simulink model "pt8612pll_2"  (Simulink 5.0)
settings: Solver=ode45  StartTime=0.0  StopTime=100  RelTol=1e-8  AbsTol=1e-11
values from neighbouring files (symbols this model uses):
  C = 680e-9    (= 6.8e-07)    [PT8612PLLinit.m]    (also in PT8612PLLinit_2.m; PT8612PLLinit_3.m; PT8612PLLinit_4.m; colorimetry_rom.m = [[CrCgCb(1) 0 0];[0 CrCgCb(2) 0];[0 0 CrCgCb(3)]])
  fvcxo = 148.5e6/1.001    (= 148351648.352)    [PT8612PLLinit.m]    (also in PT8612PLLinit_2.m; PT8612PLLinit_3.m; PT8612PLLinit_4.m)
  Gi = 1/32    (= 0.03125)    [PT8612PLLinit.m]    (also in PT8612PLLinit_2.m = 0.05)
  Gp = 1/4    (= 0.25)    [PT8612PLLinit.m]    (also in PT8612PLLinit_2.m = 0.025; PT8612PLLinit_4.m = 256)
  Kvcxo = 90e-6    (= 9e-05)    [PT8612PLLinit.m]    (also in PT8612PLLinit_2.m; PT8612PLLinit_3.m; PT8612PLLinit_4.m)
  Nbit = 12    [PT8612PLLinit_2.m]    (also in PT8612PLLinit_3.m)
  R = 100e3    (= 100000)    [PT8612PLLinit.m]    (also in PT8612PLLinit_2.m = 220000; PT8612PLLinit_3.m = 82000; PT8612PLLinit_4.m = 200000; combi_signal.m = [R;ones(red_heigth,spl)])
  Tds = 8/fvcxo    (= 5.39259259259e-08)    [PT8612PLLinit_2.m]    (also in PT8612PLLinit_3.m; PT8612PLLinit_4.m)
  Vcc = 3.3    [PT8612PLLinit_2.m]    (also in PT8612PLLinit_3.m; PT8612PLLinit_4.m)
libraries: simulink x2
settings Model: LastModifiedBy=thh

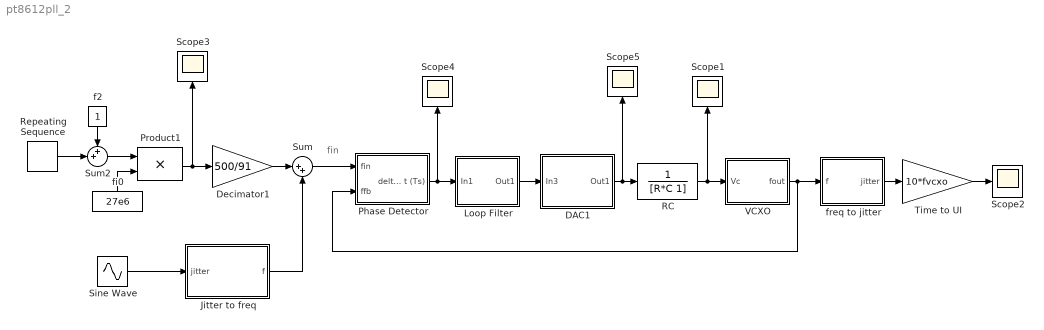
== system pt8612pll_2 ==
  note: fin
  DAC1 : Subsystem
  Decimator1 : Gain  Gain=500/91  SaturateOnIntegerOverflow=on
  Jitter to freq : Subsystem
  Loop Filter : Subsystem
  Phase Detector : Subsystem
  Product1 : Product  SaturateOnIntegerOverflow=on
  RC : TransferFcn  Denominator=[R*C 1]
  Repeating Sequence : simulink/Sources/Repeating Sequence  rep_seq_t=[0 1 1 1000]  rep_seq_y=[1 1 0 0]*1e-9
  Scope{1..5} (5 alike) : Scope
      Scope1 settings: Orientation=up  TimeRange=10  YMin=-0.35  YMax=0.2
      Scope2 settings: TimeRange=10  YMin=1.48  YMax=1.56  SaveName=ScopeData3
      Scope3 settings: Orientation=up  YMin=5.55112e-017  YMax=1.9  SaveName=ScopeData4
      Scope4 settings: Orientation=up  TimeRange=10  YMin=-0.5  YMax=0.5
      Scope5 settings: Orientation=up  TimeRange=10  YMin=-0.35  YMax=0.2  SaveName=ScopeData5
  Sine Wave : Sin  Amplitude=1e-9  Frequency=100  SampleTime=0
  Sum : Sum  Inputs=|++  SaturateOnIntegerOverflow=on
  Sum2 : Sum  Inputs=++|  SaturateOnIntegerOverflow=on
  Time to UI : Gain  Gain=10*fvcxo  SaturateOnIntegerOverflow=on
  VCXO : Subsystem
  f2 : Constant  Orientation=down
  fi0 : Constant  Orientation=up  Value=27e6
  freq to jitter : Subsystem
  wires:
  Phase Detector/1(delta t (Ts)) -> Loop Filter/1(In1), Scope4/1
  VCXO/1(fout) -> freq to jitter/1(f), Phase Detector/2(ffb)
  Product1/1 -> Scope3/1, Decimator1/1
  f2/1 -> Sum2/1
  Sum2/1 -> Product1/1
  Repeating Sequence/1 -> Sum2/2
  Loop Filter/1(Out1) -> DAC1/1(In3)
  freq to jitter/1(jitter) -> Time to UI/1
  fi0/1 -> Product1/2
  Time to UI/1 -> Scope2/1
  Sum/1 -> Phase Detector/1(fin)
  Decimator1/1 -> Sum/1
  Jitter to freq/1(f) -> Sum/2
  Sine Wave/1 -> Jitter to freq/1(jitter)
  DAC1/1(Out1) -> RC/1, Scope5/1
  RC/1 -> VCXO/1(Vc), Scope1/1

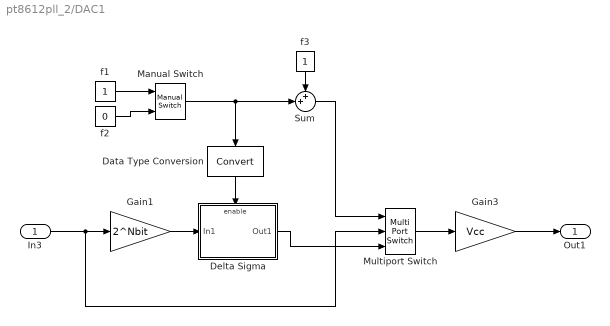
== system pt8612pll_2/DAC1 ==
  In3 : Inport
  Data Type Conversion : DataTypeConversion  Orientation=down  DataType=boolean  SaturateOnIntegerOverflow=on
  Delta Sigma : Subsystem
  Gain1 : Gain  Gain=2^Nbit  SaturateOnIntegerOverflow=on
  Gain3 : Gain  Gain=Vcc  SaturateOnIntegerOverflow=on
  Manual Switch : simulink/Signal Routing/Manual Switch  sw=0  action=0
  Multiport Switch : MultiPortSwitch  Inputs=2  SaturateOnIntegerOverflow=on
  Sum : Sum  Inputs=++|  SaturateOnIntegerOverflow=on
  f1 : Constant
  f2 : Constant  Value=0
  f3 : Constant  Orientation=down
  Out1 : Outport
  wires:
  Delta Sigma/1(Out1) -> Multiport Switch/3
  f3/1 -> Sum/1
  Sum/1 -> Multiport Switch/1
  Gain3/1 -> Out1/1
  Gain1/1 -> Delta Sigma/1(In1)
  Multiport Switch/1 -> Gain3/1
  f2/1 -> Manual Switch/2
  f1/1 -> Manual Switch/1
  Manual Switch/1 -> Sum/2, Data Type Conversion/1
  In3/1 -> Multiport Switch/2, Gain1/1
  Data Type Conversion/1 -> Delta Sigma/Enable

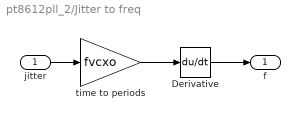
== system pt8612pll_2/Jitter to freq ==
  jitter : Inport
  Derivative : Derivative
  time to periods : Gain  Gain=fvcxo  SaturateOnIntegerOverflow=on
  f : Outport
  wires:
  time to periods/1 -> Derivative/1
  jitter/1 -> time to periods/1
  Derivative/1 -> f/1

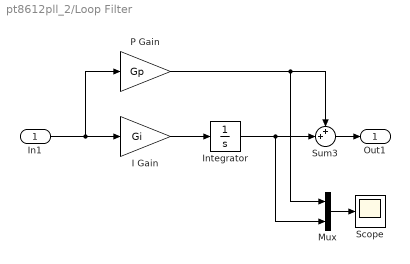
== system pt8612pll_2/Loop Filter ==
  In1 : Inport
  I Gain : Gain  Gain=Gi  SaturateOnIntegerOverflow=on
  Integrator : Integrator
  Mux : Mux  Inputs=2
  P Gain : Gain  Gain=Gp  SaturateOnIntegerOverflow=on
  Scope : Scope
      settings: YMin=0  YMax=0.85  SaveName=ScopeData2
  Sum3 : Sum  Inputs=++|  SaturateOnIntegerOverflow=on
  Out1 : Outport
  wires:
  I Gain/1 -> Integrator/1
  P Gain/1 -> Sum3/1, Mux/1
  In1/1 -> I Gain/1, P Gain/1
  Sum3/1 -> Out1/1
  Mux/1 -> Scope/1
  Integrator/1 -> Sum3/2, Mux/2

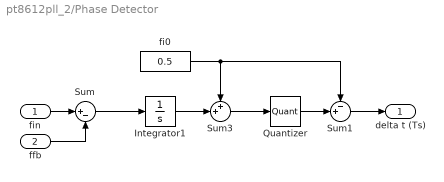
== system pt8612pll_2/Phase Detector ==
  fin : Inport
  ffb : Inport  Port=2
  Integrator1 : Integrator
  Quantizer : Quantizer  QuantizationInterval=1
  Sum : Sum  Inputs=|+-  SaturateOnIntegerOverflow=on
  Sum1 : Sum  Inputs=-+|  SaturateOnIntegerOverflow=on
  Sum3 : Sum  Inputs=++|  SaturateOnIntegerOverflow=on
  fi0 : Constant  Value=0.5
  delta t (Ts) : Outport
  wires:
  Sum/1 -> Integrator1/1
  fin/1 -> Sum/1
  ffb/1 -> Sum/2
  Sum3/1 -> Quantizer/1
  Integrator1/1 -> Sum3/2
  Quantizer/1 -> Sum1/2
  Sum1/1 -> delta t (Ts)/1
  fi0/1 -> Sum3/1, Sum1/1

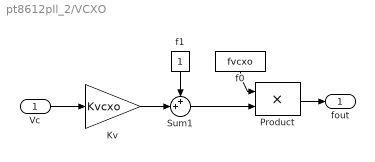
== system pt8612pll_2/VCXO ==
  Vc : Inport
  Kv : Gain  Gain=Kvcxo  SaturateOnIntegerOverflow=on
  Product : Product  SaturateOnIntegerOverflow=on
  Sum1 : Sum  Inputs=++|  SaturateOnIntegerOverflow=on
  f0 : Constant  Orientation=down  Value=fvcxo
  f1 : Constant  Orientation=down
  fout : Outport
  wires:
  f0/1 -> Product/1
  f1/1 -> Sum1/1
  Sum1/1 -> Product/2
  Kv/1 -> Sum1/2
  Vc/1 -> Kv/1
  Product/1 -> fout/1

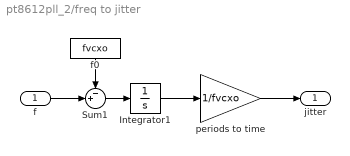
== system pt8612pll_2/freq to jitter ==
  f : Inport
  Integrator1 : Integrator
  Sum1 : Sum  Inputs=-+|  SaturateOnIntegerOverflow=on
  f0 : Constant  Orientation=down  Value=fvcxo
  periods to time : Gain  Gain=1/fvcxo  SaturateOnIntegerOverflow=on
  jitter : Outport
  wires:
  Integrator1/1 -> periods to time/1
  Sum1/1 -> Integrator1/1
  f0/1 -> Sum1/1
  f/1 -> Sum1/2
  periods to time/1 -> jitter/1

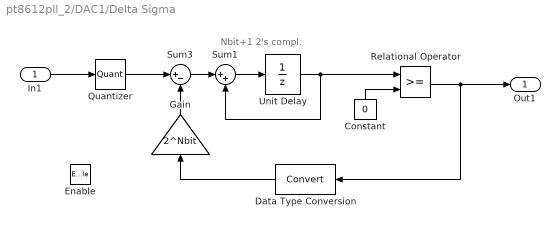
== system pt8612pll_2/DAC1/Delta Sigma ==
  note: Nbit+1 2's compl.
  In1 : Inport
  Enable : EnablePort  ZeroCross=off
  Constant : Constant  Orientation=up  Value=0
  Data Type Conversion : DataTypeConversion  Orientation=left  SaturateOnIntegerOverflow=on
  Gain : Gain  Orientation=up  Gain=2^Nbit  SaturateOnIntegerOverflow=on
  Quantizer : Quantizer  QuantizationInterval=1
  Relational Operator : RelationalOperator
  Sum1 : Sum  Inputs=|++  SaturateOnIntegerOverflow=on
  Sum3 : Sum  Inputs=|+-  SaturateOnIntegerOverflow=on
  Unit Delay : UnitDelay  SampleTime=Tds
  Out1 : Outport
  wires:
  Gain/1 -> Sum3/2
  Quantizer/1 -> Sum3/1
  In1/1 -> Quantizer/1
  Data Type Conversion/1 -> Gain/1
  Sum3/1 -> Sum1/1
  Sum1/1 -> Unit Delay/1
  Relational Operator/1 -> Out1/1, Data Type Conversion/1
  Constant/1 -> Relational Operator/2
  Unit Delay/1 -> Relational Operator/1, Sum1/2
